simulink model "modello_completo_simulink2020"  (R2020a)
settings: Solver=VariableStepAuto  StartTime=0.0  StopTime=200  RelTol=1e-3
values from neighbouring files (symbols this model uses):
  a = 0.35    [data.m]    (also in geodetic2nedS.m = 6378137)
  a1 = rho * D^4 * alpha1    (= 0.000388302366464)    [data.m]
  a2 = -rho * D^3 * alpha2 * (1 - omega)    (= 0.0037030698432)    [data.m]
  AHRS_bias = [0 0 0]    [data.m]
  AHRS_sample_time = 1/50    (= 0.02)    [data.m]
  AHRS_var = ([1 1 2] * pi/180).^2    [data.m]
  alpha1 = 0.0113    [data.m]
  alpha2 = -0.0091    [data.m]
  c = son2(1)    [Sonar_id.m]    (also in data.m = 0.19)
  current = [seaCurrent; 0; 0; 0]    [data.m]
  D = 0.076    [data.m]
  dead_zone_limit = 31.5    [data.m]
  DVL_sample_t = 1/12    (= 0.0833333333333)    [data.m]
  DVL_var1 = 0.005^2    (= 2.5e-05)    [data.m]
  DVL_var2 = 0.015^2    (= 0.000225)    [data.m]
  DVL_var3 = 0.023^2    (= 0.000529)    [data.m]
  gps_sample_t = 1    [data.m]
  H = eye(3)    [data.m]    (also in navigation_data.m)
  IMU_sample_time = 1/100    (= 0.01)    [data.m]
  initial = []    [data.m]
  INSP = unicode2native(inspectionDirection)    [data.m]
  Ki_bodypos1 = 0    [parametri_PID.m]
  Ki_bodypos2 = 0    [parametri_PID.m]
  Ki_bodypos3 = 0    [parametri_PID.m]
  Ki_bodypos4 = 0    [parametri_PID.m]
  Ki_bodypos5 = 0    [parametri_PID.m]
  Ki_depth1 = 0    [parametri_PID.m]
  Ki_depth2 = 0    [parametri_PID.m]
  Ki_depth3 = 0    [parametri_PID.m]
  Ki_depth4 = 0    [parametri_PID.m]
  Ki_depth5 = 0    [parametri_PID.m]
  Ki_latvel1 = 0    [parametri_PID.m]
  Ki_latvel2 = 0    [parametri_PID.m]
  Ki_latvel3 = 0    [parametri_PID.m]
  Ki_latvel4 = 0    [parametri_PID.m]
  Ki_latvel5 = 0    [parametri_PID.m]
  Ki_P1 = 0    [parametri_PID.m]
  Ki_P2 = 0    [parametri_PID.m]
  Ki_P3 = 0    [parametri_PID.m]
  Ki_P4 = 0    [parametri_PID.m]
  Ki_P5 = 0    [parametri_PID.m]
  Ki_R1 = 0    [parametri_PID.m]
  Ki_R2 = 0    [parametri_PID.m]
  Ki_R3 = 0    [parametri_PID.m]
  Ki_R4 = 0    [parametri_PID.m]
  Ki_R5 = 0    [parametri_PID.m]
  Ki_rel_or1 = 0    [parametri_PID.m]
  Ki_rel_or2 = 0    [parametri_PID.m]
  Ki_rel_or3 = 0    [parametri_PID.m]
  Ki_rel_or4 = 0    [parametri_PID.m]
  Ki_rel_or5 = 0    [parametri_PID.m]
  Ki_reldist1 = 0    [parametri_PID.m]
  Ki_reldist2 = 0    [parametri_PID.m]
  Ki_reldist3 = 0    [parametri_PID.m]
  Ki_reldist4 = 0    [parametri_PID.m]
  Ki_reldist5 = 0    [parametri_PID.m]
  Ki_surge1 = 0    [parametri_PID.m]
  Ki_surge2 = 0    [parametri_PID.m]
  Ki_surge3 = 0    [parametri_PID.m]
  Ki_surge4 = 0    [parametri_PID.m]
  Ki_surge5 = 0    [parametri_PID.m]
  Ki_yaw1 = 0    [parametri_PID.m]
  Ki_yaw2 = 0    [parametri_PID.m]
  Ki_yaw3 = 0    [parametri_PID.m]
  Ki_yaw4 = 0    [parametri_PID.m]
  Ki_yaw5 = 0    [parametri_PID.m]
  Kp_bodypos1 = 0    [parametri_PID.m]
  Kp_bodypos2 = 2    [parametri_PID.m]
  Kp_bodypos3 = 2    [parametri_PID.m]
  Kp_bodypos4 = 2    [parametri_PID.m]
  Kp_bodypos5 = 2    [parametri_PID.m]
  Kp_depth1 = 0    [parametri_PID.m]
  Kp_depth2 = 2    [parametri_PID.m]
  Kp_depth3 = 2    [parametri_PID.m]
  Kp_depth4 = 2    [parametri_PID.m]
  Kp_depth5 = 2    [parametri_PID.m]
  Kp_latvel1 = 0    [parametri_PID.m]
  Kp_latvel2 = 2    [parametri_PID.m]
  Kp_latvel3 = 2    [parametri_PID.m]
  Kp_latvel4 = 2    [parametri_PID.m]
  Kp_latvel5 = 2    [parametri_PID.m]
  Kp_P1 = 0    [parametri_PID.m]
  Kp_P2 = 2    [parametri_PID.m]
  Kp_P3 = 2    [parametri_PID.m]
  Kp_P4 = 2    [parametri_PID.m]
  Kp_P5 = 2    [parametri_PID.m]
  Kp_R1 = 0    [parametri_PID.m]
  Kp_R2 = 2    [parametri_PID.m]
  Kp_R3 = 2    [parametri_PID.m]
  Kp_R4 = 2    [parametri_PID.m]
  Kp_R5 = 2    [parametri_PID.m]
  Kp_rel_or1 = 0    [parametri_PID.m]
  Kp_rel_or2 = 2    [parametri_PID.m]
  Kp_rel_or3 = 2    [parametri_PID.m]
  Kp_rel_or4 = 2    [parametri_PID.m]
  Kp_rel_or5 = 2    [parametri_PID.m]
  Kp_reldist1 = 0    [parametri_PID.m]
  Kp_reldist2 = 2    [parametri_PID.m]
  Kp_reldist3 = 2    [parametri_PID.m]
  Kp_reldist4 = 2    [parametri_PID.m]
  Kp_reldist5 = 2    [parametri_PID.m]
  Kp_surge1 = 0    [parametri_PID.m]
  Kp_surge2 = 2    [parametri_PID.m]
  Kp_surge3 = 2    [parametri_PID.m]
  Kp_surge4 = 2    [parametri_PID.m]
  Kp_surge5 = 2    [parametri_PID.m]
  Kp_yaw1 = 0.6*6    (= 3.6)    [parametri_PID.m]
  Kp_yaw2 = 2    [parametri_PID.m]
  Kp_yaw3 = 2    [parametri_PID.m]
  Kp_yaw4 = 2    [parametri_PID.m]
  Kp_yaw5 = 2    [parametri_PID.m]
  M = M_rb + M_a    [Masse.m]
  M_inv = inv(M)    [Masse.m]
  n_max = 340    [data.m]
  num_cycle = 5    [data.m]    (also in navigation_data.m)
  omega = 0.1    [data.m]
  plot_smpl = 0.1    [data.m]
  ps_sample_t = 0.02    [data.m]
  ps_var = (5000/3)^2    (= 2777777.77778)    [data.m]
  pylonCenter = [ 43.723046 ... (first row only)    [missionB.m]
  ... (+4 more)
undefined symbols (not defined in the file or in its folder): DiscIntNeverNeededParam, s_data
libraries: simulink x3
(part 3 of 5)

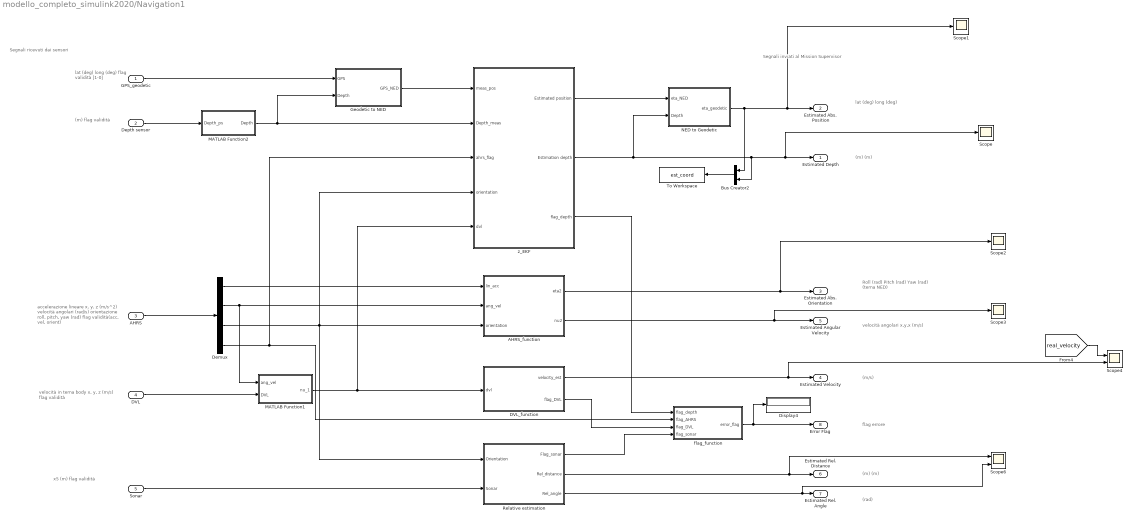
== system modello_completo_simulink2020/Navigation1 ==
  note: (m/s)
  note: (rad)
  note: (m)
      | (m)
  note: (m)
      | flag validità
  note: velocità in terna body x, y, z (m/s)
      | flag validità
  note: Segnali ricevuti dai sensori
  note: flag errore
  note: accelerazione lineare x, y, z (m/s^2)
      | velocità angolari (rad/s)
      | orientazione roll, pitch, yaw (rad)
      | flag validità(acc, vel, orient)
  note: velocità angolari x,y,x (m/s)
  note: lat     (deg)
      |  long  (deg)
  note: (m)
      | (m)
  note: Roll (rad)
      | Pitch (rad)
      | Yaw (rad)
      | (terna NED)
  note: x5
      | (m)
      | flag validità
  note: Segnali inviati al Mission Supervisor
  note: lat     (deg)
      |  long  (deg)
      | flag validità [1-0]
  GPS_geodetic : Inport  PortDimensions=3
  Depth sensor : Inport  Port=2  PortDimensions=2
  AHRS : Inport  Port=3  PortDimensions=12
  DVL : Inport  Port=4  PortDimensions=4
  Sonar : Inport  Port=5
  AHRS_function : MATLAB Function  TreatAsAtomicUnit=on
  Bus Creator2 : BusCreator  Inputs=2
  DVL_function : MATLAB Function  TreatAsAtomicUnit=on
  Demux : Demux  Outputs=[3 3 3 3]
  Display4 : Display
  Geodetic to NED : Subsystem
  MATLAB Function1 : MATLAB Function  TreatAsAtomicUnit=on  SystemSampleTime=DVL_sample_t
  MATLAB Function2 : MATLAB Function  TreatAsAtomicUnit=on
  NED to Geodetic : Subsystem
  Relative estimation : Subsystem
  Scope{,1..3} (4 alike) : Scope
  Scope4 : Scope  NumInputPorts=2
  Scope6 : Scope  NumInputPorts=2
  To Workspace : ToWorkspace  VariableName=est_coord  SampleTime=-1
  flag_function : MATLAB Function  TreatAsAtomicUnit=on  SystemSampleTime=1/200
  z_EKF : Subsystem
  Estimated Depth : Outport
  Estimated Abs. Position : Outport  Port=2
  Estimated Abs. Orientation : Outport  Port=3
  Estimated Velocity : Outport  Port=4
  Estimated Angular Velocity : Outport  Port=5
  Estimated Rel. Distance : Outport  Port=6
  Estimated Rel. Angle : Outport  Port=7
  Error Flag : Outport  Port=8
  wires:
  z_EKF/1(Estimated position) -> NED to Geodetic/1(eta_NED)
  [real_velocity] -> Scope4/1
  Relative estimation/1(Flag_sonar) -> flag_function/4(flag_sonar)
  Bus Creator2/1 -> To Workspace/1
  Demux/4 -> z_EKF/3(ahrs_flag), flag_function/2(flag_AHRS)
  MATLAB Function2/1(Depth) -> Geodetic to NED/2(Depth), z_EKF/2(Depth_meas)
  NED to Geodetic/1(eta_geodetic) -> Bus Creator2/1, Scope1/1, Estimated Abs. Position/1
  z_EKF/3(flag_depth) -> flag_function/1(flag_depth)
  flag_function/1(error_flag) -> Display4/1, Error Flag/1
  AHRS_function/1(eta2) -> Scope2/1, Estimated Abs. Orientation/1
  DVL_function/1(velocity_est) -> Scope4/2, Estimated Velocity/1
  AHRS/1 -> Demux/1
  Sonar/1 -> Relative estimation/2(Sonar)
  Demux/2 -> MATLAB Function1/1(ang_vel), AHRS_function/2(ang_vel)
  Relative estimation/2(Rel_distance) -> Scope6/1, Estimated Rel. Distance/1
  MATLAB Function1/1(nu_1) -> z_EKF/5(dvl), DVL_function/1(dvl)
  Geodetic to NED/1(GPS_NED) -> z_EKF/1(meas_pos)
  z_EKF/2(Estimation depth) -> NED to Geodetic/2(Depth), Bus Creator2/2, Scope/1, Estimated Depth/1
  Relative estimation/3(Rel_angle) -> Scope6/2, Estimated Rel. Angle/1
  GPS_geodetic/1 -> Geodetic to NED/1(GPS)
  DVL_function/2(flag_DVL) -> flag_function/3(flag_DVL)
  Depth sensor/1 -> MATLAB Function2/1(Depth_ps)
  DVL/1 -> MATLAB Function1/2(DVL)
  Demux/3 -> z_EKF/4(orientation), AHRS_function/3(orientation), Relative estimation/1(Orientation)
  AHRS_function/2(nu2) -> Scope3/1, Estimated Angular Velocity/1
  Demux/1 -> AHRS_function/1(lin_acc)

== system modello_completo_simulink2020/Vehicle Model ==
  note: 3x1 (m/s^2),
      | 3x1 (rad/s^2)
  note: 3x1 (m/s),
      | 3x1 (rad/s)
  note: lat (deg)
      | long (deg)
      | prof. (m),
      | roll (rad),
      | pitch (rad),
      | yaw (rad)
  note: 3x1 (m/s),
      | 3x1 (rad/s)
  Desired Thruster Rot. Speed : Inport
  Add : Sum  Inputs=+-
  Constant : Constant  Value=[100; -100; 0; 0; 0; 0; 0]
  Current : Constant  Value=current
  Demux : Demux
  MATLAB Function : MATLAB Function  TreatAsAtomicUnit=on
  Manual (by dashboard sensors) : Subsystem
  Manual Switch : ManualSwitch  CurrentSetting=0
  Manual Switch1 : ManualSwitch
  Model Vehicle : Subsystem
      mask Display: image('$imagefile'); % Use "Edit Image" on toolstrip to change.
  Scope : Scope
  Scope1 : Scope
  Thrusters : Subsystem
      mask Display: image('$imagefile'); % Use "Edit Image" on toolstrip to change.
  Position : Outport
  Velocity_NED : Outport  Port=2
  Acceleration : Outport  Port=3
  Velocity_body : Outport  Port=4
  wires:
  Demux/3 -> Velocity_body/1, Add/2  "ni"
  Model Vehicle/1(Out1) -> Demux/1
  Demux/1 -> Thrusters/2(eta), MATLAB Function/1(eta), Position/1, Scope/1  "eta"
  Desired Thruster Rot. Speed/1 -> Manual Switch/2
  Manual Switch/1 -> Thrusters/1(des rot)
  Current/1 -> MATLAB Function/2(current)
  Demux/2 -> Velocity_NED/1  "eta_dot"
  Demux/4 -> Acceleration/1  "ni_dot"
  MATLAB Function/1(ni_c) -> Model Vehicle/2(ni_current), Add/1
  Add/1 -> Thrusters/3(ni)
  Constant/1 -> Manual Switch/1
  Thrusters/1(tau) -> Manual Switch1/2, Scope1/1
  Manual (by dashboard sensors)/1(y) -> Manual Switch1/1
  Manual Switch1/1 -> Model Vehicle/1(tau)

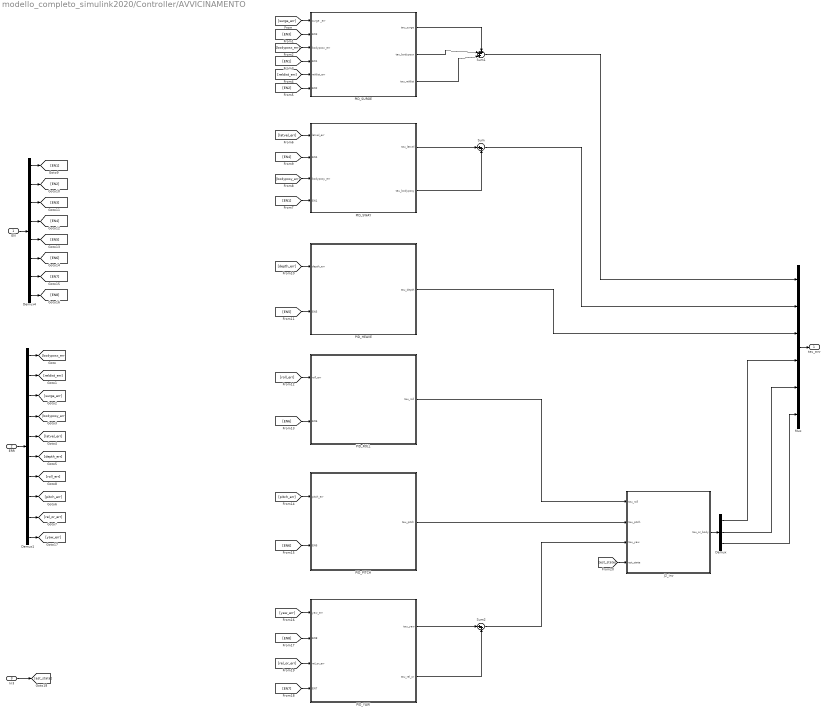
== system modello_completo_simulink2020/Controller/AVVICINAMENTO ==
  EN : Inport
  ERR : Inport  Port=2
  In3 : Inport  Port=3
  Demux : Demux  Outputs=3
  Demux1 : Demux  Outputs=10
  Demux4 : Demux  Outputs=8
  J2_inv : MATLAB Function  TreatAsAtomicUnit=on
  Mux : Mux  Inputs=6
  PID_HEAVE : Subsystem
  PID_PITCH : Subsystem
  "PID_ROLL " : Subsystem
  PID_SURGE : Subsystem
  PID_SWAY : Subsystem
  PID_YAW : Subsystem
  Sum : Sum  Inputs=|++
  Sum1 : Sum  Inputs=+++|
  Sum2 : Sum  Inputs=|++
  tau_avv : Outport
  wires:
  EN/1 -> Demux4/1
  ERR/1 -> Demux1/1
  Demux4/1 -> [EN1]
  Demux4/2 -> [EN2]
  Demux4/3 -> [EN3]
  Demux4/4 -> [EN4]
  Demux4/5 -> [EN5]
  Demux4/6 -> [EN6]
  Demux4/7 -> [EN7]
  Demux4/8 -> [EN8]
  Demux1/1 -> [bodyposx_err]
  Demux1/2 -> [reldist_err]
  Demux1/3 -> [surge_err]
  Demux1/4 -> [bodyposy_err]
  Demux1/5 -> [latvel_err]
  Demux1/6 -> [depth_err]
  Demux1/7 -> [roll_err]
  Demux1/8 -> [pitch_err]
  Demux1/9 -> [rel_or_err]
  Demux1/10 -> [yaw_err]
  [surge_err] -> PID_SURGE/1(surge _err)
  [EN3] -> PID_SURGE/2(EN3)
  [bodyposx_err] -> PID_SURGE/3(bodyposx_err)
  [EN1] -> PID_SURGE/4(EN1)
  [reldist_err] -> PID_SURGE/5(reldist_err)
  [EN2] -> PID_SURGE/6(EN2)
  [latvel_err] -> PID_SWAY/1(latvel_err)
  [bodyposy_err] -> PID_SWAY/3(bodyposy_err)
  [depth_err] -> PID_HEAVE/1(depth_err)
  [roll_err] -> "PID_ROLL "/1(roll_err)
  [pitch_err] -> PID_PITCH/1(pitch_err)
  [EN6] -> PID_PITCH/2(EN6)
  [yaw_err] -> PID_YAW/1(yaw_err)
  [EN4] -> PID_SWAY/2(EN4)
  [EN1] -> PID_SWAY/4(EN1)
  [EN5] -> PID_HEAVE/2(EN5)
  [EN6] -> "PID_ROLL "/2(EN6)
  [EN8] -> PID_YAW/2("EN8 ")
  [EN7] -> PID_YAW/4(EN7)
  [rel_or_err] -> PID_YAW/3(rel_or_err)
  PID_HEAVE/1(tau_depth) -> Mux/3
  PID_SURGE/1(tau_surge) -> Sum1/1
  Mux/1 -> tau_avv/1
  Sum1/1 -> Mux/1
  Sum/1 -> Mux/2
  PID_YAW/1(tau_yaw) -> Sum2/1
  PID_SWAY/2(tau_bodyposy) -> Sum/2
  PID_SURGE/3(tau_reldist) -> Sum1/3
  PID_SURGE/2(tau_bodyposx) -> Sum1/2
  PID_YAW/2(tau_rel_or) -> Sum2/2
  PID_SWAY/1(tau_latvel) -> Sum/1
  Demux/2 -> Mux/5
  PID_PITCH/1(tau_pitch) -> J2_inv/2(tau_pitch)
  J2_inv/1(tau_or_body) -> Demux/1
  Demux/3 -> Mux/6
  "PID_ROLL "/1(tau_roll) -> J2_inv/1(tau_roll)
  Demux/1 -> Mux/4
  [est_state] -> J2_inv/4(est_state)
  Sum2/1 -> J2_inv/3(tau_yaw)
  In3/1 -> [est_state]

== system modello_completo_simulink2020/Controller/GEODETIC2NED2 ==
  Estimated Abs. Postion : Inport  Unit=deg  PortDimensions=2
  GEODETIC2NED1 : Subsystem
  Out1 : Outport
  wires:
  GEODETIC2NED1/1(Out1) -> Out1/1
  Estimated Abs. Postion/1 -> GEODETIC2NED1/1(In1)

== system modello_completo_simulink2020/Controller/GEODETIC2NED3 ==
  In1 : Inport
  Demux2 : Demux  Outputs=2
  GEODETIC2NED : Subsystem
  Out1 : Outport
  wires:
  Demux2/2 -> GEODETIC2NED/2(lon)
  GEODETIC2NED/1(Out1) -> Out1/1
  Demux2/1 -> GEODETIC2NED/1(lat)
  In1/1 -> Demux2/1

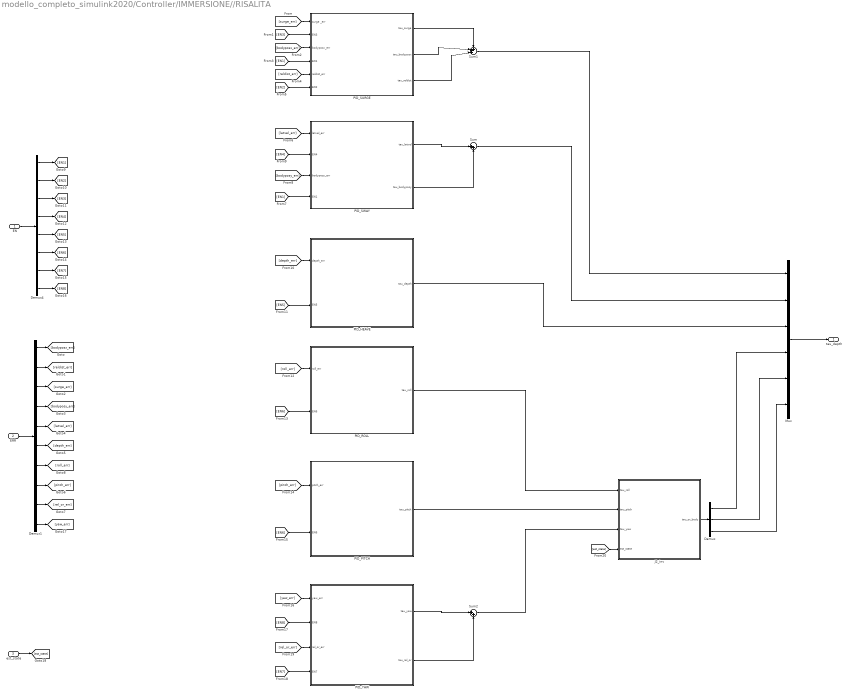
== system modello_completo_simulink2020/Controller/IMMERSIONE//RISALITA ==
  EN : Inport
  ERR : Inport  Port=2
  est_state : Inport  Port=3
  Demux : Demux  Outputs=3
  Demux1 : Demux  Outputs=10
  Demux4 : Demux  Outputs=8
  J2_inv : MATLAB Function  TreatAsAtomicUnit=on
  Mux : Mux  Inputs=6
  PID_HEAVE : Subsystem
  PID_PITCH : Subsystem
  "PID_ROLL " : Subsystem
  PID_SURGE : Subsystem
  PID_SWAY : Subsystem
  PID_YAW : Subsystem
  Sum : Sum  Inputs=|++
  Sum1 : Sum  Inputs=+++|
  Sum2 : Sum  Inputs=|++
  tau_depth : Outport
  wires:
  EN/1 -> Demux4/1
  ERR/1 -> Demux1/1
  Demux4/1 -> [EN1]
  Demux4/2 -> [EN2]
  Demux4/3 -> [EN3]
  Demux4/4 -> [EN4]
  Demux4/5 -> [EN5]
  Demux4/6 -> [EN6]
  Demux4/7 -> [EN7]
  Demux4/8 -> [EN8]
  Demux1/1 -> [bodyposx_err]
  Demux1/2 -> [reldist_err]
  Demux1/3 -> [surge_err]
  Demux1/4 -> [bodyposy_err]
  Demux1/5 -> [latvel_err]
  Demux1/6 -> [depth_err]
  Demux1/7 -> [roll_err]
  Demux1/8 -> [pitch_err]
  Demux1/9 -> [rel_or_err]
  Demux1/10 -> [yaw_err]
  [surge_err] -> PID_SURGE/1(surge _err)
  [EN3] -> PID_SURGE/2(EN3)
  [bodyposx_err] -> PID_SURGE/3(bodyposx_err)
  [EN1] -> PID_SURGE/4(EN1)
  [reldist_err] -> PID_SURGE/5(reldist_err)
  [EN2] -> PID_SURGE/6(EN2)
  [latvel_err] -> PID_SWAY/1(latvel_err)
  [bodyposy_err] -> PID_SWAY/3(bodyposy_err)
  [depth_err] -> PID_HEAVE/1(depth_err)
  [roll_err] -> "PID_ROLL "/1(roll_err)
  [pitch_err] -> PID_PITCH/1(pitch_err)
  [EN6] -> PID_PITCH/2(EN6)
  [yaw_err] -> PID_YAW/1(yaw_err)
  [EN4] -> PID_SWAY/2(EN4)
  [EN1] -> PID_SWAY/4(EN1)
  [EN5] -> PID_HEAVE/2(EN5)
  [EN6] -> "PID_ROLL "/2(EN6)
  [EN8] -> PID_YAW/2("EN8 ")
  [EN7] -> PID_YAW/4(EN7)
  [rel_or_err] -> PID_YAW/3(rel_or_err)
  PID_HEAVE/1(tau_depth) -> Mux/3
  PID_SURGE/1(tau_surge) -> Sum1/1
  Mux/1 -> tau_depth/1
  Sum1/1 -> Mux/1
  Sum/1 -> Mux/2
  PID_YAW/1(tau_yaw) -> Sum2/1
  PID_SWAY/2(tau_bodyposy) -> Sum/2
  PID_SURGE/3(tau_reldist) -> Sum1/3
  PID_SURGE/2(tau_bodyposx) -> Sum1/2
  PID_YAW/2(tau_rel_or) -> Sum2/2
  PID_SWAY/1(tau_latvel) -> Sum/1
  Demux/2 -> Mux/5
  [est_state] -> J2_inv/4(est_state)
  "PID_ROLL "/1(tau_roll) -> J2_inv/1(tau_roll)
  Demux/3 -> Mux/6
  Demux/1 -> Mux/4
  PID_PITCH/1(tau_pitch) -> J2_inv/2(tau_pitch)
  Sum2/1 -> J2_inv/3(tau_yaw)
  J2_inv/1(tau_or_body) -> Demux/1
  est_state/1 -> [est_state]

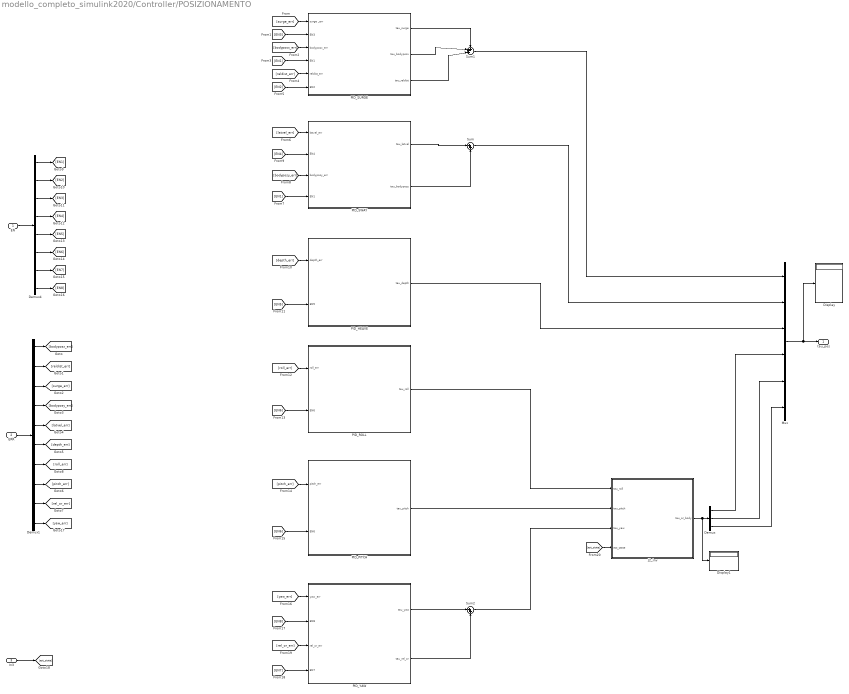
== system modello_completo_simulink2020/Controller/POSIZIONAMENTO ==
  EN : Inport
  ERR : Inport  Port=2
  In3 : Inport  Port=3
  Demux : Demux  Outputs=3
  Demux1 : Demux  Outputs=10
  Demux4 : Demux  Outputs=8
  Display : Display
  Display1 : Display
  J2_inv : MATLAB Function  TreatAsAtomicUnit=on
  Mux : Mux  Inputs=6
  PID_HEAVE : Subsystem
  PID_PITCH : Subsystem
  "PID_ROLL " : Subsystem
  PID_SURGE : Subsystem
  PID_SWAY : Subsystem
  PID_YAW : Subsystem
  Sum : Sum  Inputs=|++
  Sum1 : Sum  Inputs=+++|
  Sum2 : Sum  Inputs=|++
  tau_pos : Outport
  wires:
  PID_SWAY/1(tau_latvel) -> Sum/1
  PID_YAW/2(tau_rel_or) -> Sum2/2
  PID_SURGE/2(tau_bodyposx) -> Sum1/2
  PID_SURGE/3(tau_reldist) -> Sum1/3
  PID_SWAY/2(tau_bodyposy) -> Sum/2
  PID_YAW/1(tau_yaw) -> Sum2/1
  Sum/1 -> Mux/2
  Sum1/1 -> Mux/1
  Mux/1 -> Display/1, tau_pos/1
  PID_SURGE/1(tau_surge) -> Sum1/1
  PID_HEAVE/1(tau_depth) -> Mux/3
  [rel_or_err] -> PID_YAW/3(rel_or_err)
  [EN7] -> PID_YAW/4(EN7)
  [EN8] -> PID_YAW/2("EN8 ")
  [EN6] -> "PID_ROLL "/2(EN6)
  [EN5] -> PID_HEAVE/2(EN5)
  [EN1] -> PID_SWAY/4(EN1)
  [EN4] -> PID_SWAY/2(EN4)
  [yaw_err] -> PID_YAW/1(yaw_err)
  [EN6] -> PID_PITCH/2(EN6)
  [pitch_err] -> PID_PITCH/1(pitch_err)
  [roll_err] -> "PID_ROLL "/1(roll_err)
  [depth_err] -> PID_HEAVE/1(depth_err)
  [bodyposy_err] -> PID_SWAY/3(bodyposy_err)
  [latvel_err] -> PID_SWAY/1(latvel_err)
  [EN2] -> PID_SURGE/6(EN2)
  [reldist_err] -> PID_SURGE/5(reldist_err)
  [EN1] -> PID_SURGE/4(EN1)
  [bodyposx_err] -> PID_SURGE/3(bodyposx_err)
  [EN3] -> PID_SURGE/2(EN3)
  [surge_err] -> PID_SURGE/1(surge _err)
  Demux1/10 -> [yaw_err]
  Demux1/9 -> [rel_or_err]
  Demux1/8 -> [pitch_err]
  Demux1/7 -> [roll_err]
  Demux1/6 -> [depth_err]
  Demux1/5 -> [latvel_err]
  Demux1/4 -> [bodyposy_err]
  Demux1/3 -> [surge_err]
  Demux1/2 -> [reldist_err]
  Demux1/1 -> [bodyposx_err]
  Demux4/8 -> [EN8]
  Demux4/7 -> [EN7]
  Demux4/6 -> [EN6]
  Demux4/5 -> [EN5]
  Demux4/4 -> [EN4]
  Demux4/3 -> [EN3]
  Demux4/2 -> [EN2]
  Demux4/1 -> [EN1]
  ERR/1 -> Demux1/1
  EN/1 -> Demux4/1
  In3/1 -> [est_state]
  [est_state] -> J2_inv/4(est_state)
  "PID_ROLL "/1(tau_roll) -> J2_inv/1(tau_roll)
  PID_PITCH/1(tau_pitch) -> J2_inv/2(tau_pitch)
  Sum2/1 -> J2_inv/3(tau_yaw)
  J2_inv/1(tau_or_body) -> Display1/1, Demux/1
  Demux/1 -> Mux/4
  Demux/2 -> Mux/5
  Demux/3 -> Mux/6

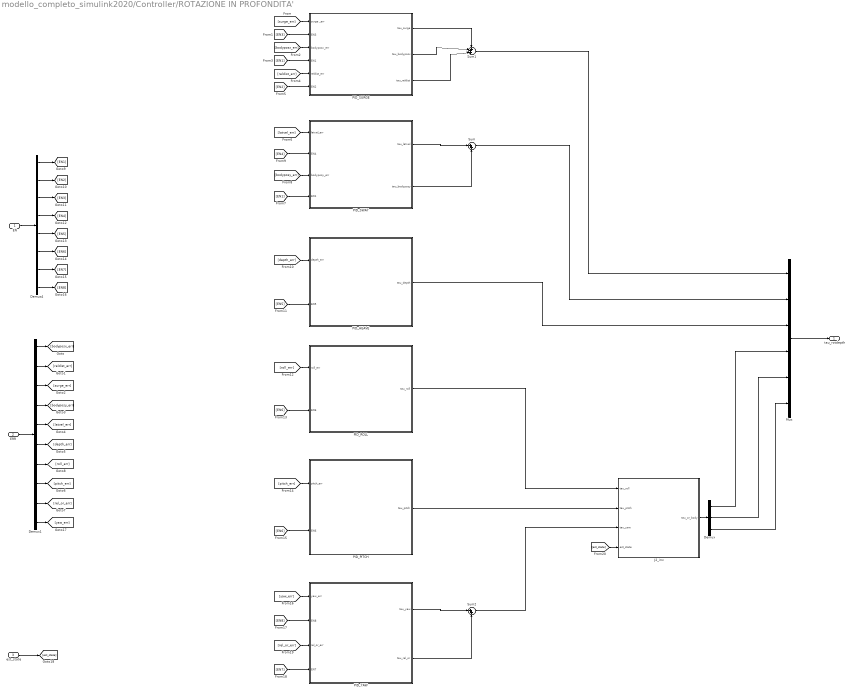
== system modello_completo_simulink2020/Controller/ROTAZIONE IN PROFONDITA' ==
  EN : Inport
  ERR : Inport  Port=2
  est_state : Inport  Port=3
  Demux : Demux  Outputs=3
  Demux1 : Demux  Outputs=10
  Demux4 : Demux  Outputs=8
  J2_inv : MATLAB Function  TreatAsAtomicUnit=on
  Mux : Mux  Inputs=6
  PID_HEAVE : Subsystem
  PID_PITCH : Subsystem
  "PID_ROLL " : Subsystem
  PID_SURGE : Subsystem
  PID_SWAY : Subsystem
  PID_YAW : Subsystem
  Sum : Sum  Inputs=|++
  Sum1 : Sum  Inputs=+++|
  Sum2 : Sum  Inputs=|++
  tau_rotdepth : Outport
  wires:
  EN/1 -> Demux4/1
  ERR/1 -> Demux1/1
  Demux4/1 -> [EN1]
  Demux4/2 -> [EN2]
  Demux4/3 -> [EN3]
  Demux4/4 -> [EN4]
  Demux4/5 -> [EN5]
  Demux4/6 -> [EN6]
  Demux4/7 -> [EN7]
  Demux4/8 -> [EN8]
  Demux1/1 -> [bodyposx_err]
  Demux1/2 -> [reldist_err]
  Demux1/3 -> [surge_err]
  Demux1/4 -> [bodyposy_err]
  Demux1/5 -> [latvel_err]
  Demux1/6 -> [depth_err]
  Demux1/7 -> [roll_err]
  Demux1/8 -> [pitch_err]
  Demux1/9 -> [rel_or_err]
  Demux1/10 -> [yaw_err]
  [surge_err] -> PID_SURGE/1(surge _err)
  [EN3] -> PID_SURGE/2(EN3)
  [bodyposx_err] -> PID_SURGE/3(bodyposx_err)
  [EN1] -> PID_SURGE/4(EN1)
  [reldist_err] -> PID_SURGE/5(reldist_err)
  [EN2] -> PID_SURGE/6(EN2)
  [latvel_err] -> PID_SWAY/1(latvel_err)
  [bodyposy_err] -> PID_SWAY/3(bodyposy_err)
  [depth_err] -> PID_HEAVE/1(depth_err)
  [roll_err] -> "PID_ROLL "/1(roll_err)
  [pitch_err] -> PID_PITCH/1(pitch_err)
  [EN6] -> PID_PITCH/2(EN6)
  [yaw_err] -> PID_YAW/1(yaw_err)
  [EN4] -> PID_SWAY/2(EN4)
  [EN1] -> PID_SWAY/4(EN1)
  [EN5] -> PID_HEAVE/2(EN5)
  [EN6] -> "PID_ROLL "/2(EN6)
  [EN8] -> PID_YAW/2("EN8 ")
  [EN7] -> PID_YAW/4(EN7)
  [rel_or_err] -> PID_YAW/3(rel_or_err)
  PID_HEAVE/1(tau_depth) -> Mux/3
  PID_SURGE/1(tau_surge) -> Sum1/1
  Mux/1 -> tau_rotdepth/1
  Sum1/1 -> Mux/1
  Sum/1 -> Mux/2
  PID_YAW/1(tau_yaw) -> Sum2/1
  PID_SWAY/2(tau_bodyposy) -> Sum/2
  PID_SURGE/3(tau_reldist) -> Sum1/3
  PID_SURGE/2(tau_bodyposx) -> Sum1/2
  PID_YAW/2(tau_rel_or) -> Sum2/2
  PID_SWAY/1(tau_latvel) -> Sum/1
  Demux/1 -> Mux/4
  Sum2/1 -> J2_inv/3(tau_yaw)
  Demux/3 -> Mux/6
  "PID_ROLL "/1(tau_roll) -> J2_inv/1(tau_roll)
  Demux/2 -> Mux/5
  [est_state] -> J2_inv/4(est_state)
  PID_PITCH/1(tau_pitch) -> J2_inv/2(tau_pitch)
  J2_inv/1(tau_or_body) -> Demux/1
  est_state/1 -> [est_state]

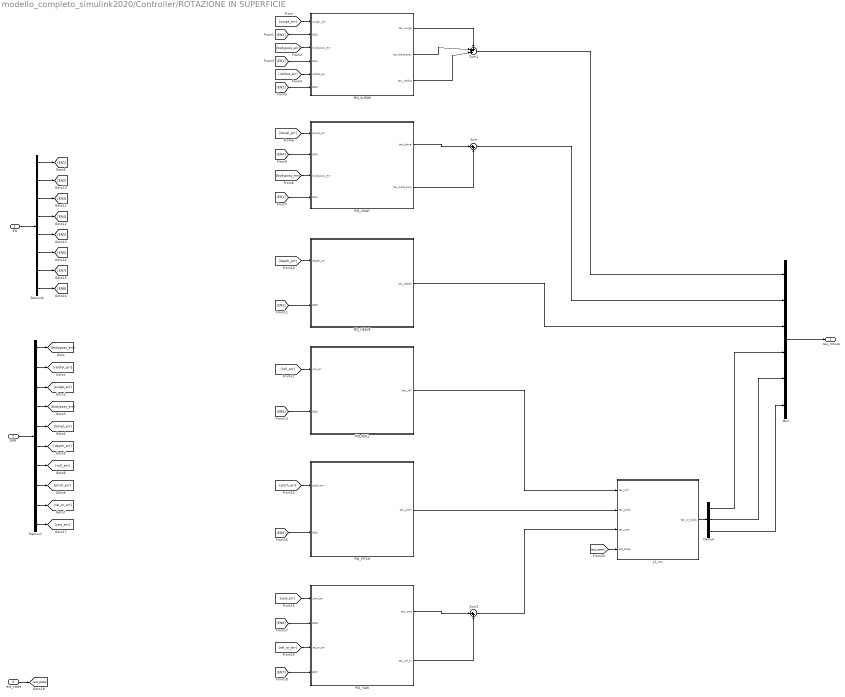
== system modello_completo_simulink2020/Controller/ROTAZIONE IN SUPERFICIE ==
  EN : Inport
  ERR : Inport  Port=2
  est_state : Inport  Port=3
  Demux : Demux  Outputs=3
  Demux1 : Demux  Outputs=10
  Demux4 : Demux  Outputs=8
  J2_inv : MATLAB Function  TreatAsAtomicUnit=on
  Mux : Mux  Inputs=6
  PID_HEAVE : Subsystem
  PID_PITCH : Subsystem
  "PID_ROLL " : Subsystem
  PID_SURGE : Subsystem
  PID_SWAY : Subsystem
  PID_YAW : Subsystem
  Sum : Sum  Inputs=|++
  Sum1 : Sum  Inputs=+++|
  Sum2 : Sum  Inputs=|++
  tau_rotsup : Outport
  wires:
  EN/1 -> Demux4/1
  ERR/1 -> Demux1/1
  Demux4/1 -> [EN1]
  Demux4/2 -> [EN2]
  Demux4/3 -> [EN3]
  Demux4/4 -> [EN4]
  Demux4/5 -> [EN5]
  Demux4/6 -> [EN6]
  Demux4/7 -> [EN7]
  Demux4/8 -> [EN8]
  Demux1/1 -> [bodyposx_err]
  Demux1/2 -> [reldist_err]
  Demux1/3 -> [surge_err]
  Demux1/4 -> [bodyposy_err]
  Demux1/5 -> [latvel_err]
  Demux1/6 -> [depth_err]
  Demux1/7 -> [roll_err]
  Demux1/8 -> [pitch_err]
  Demux1/9 -> [rel_or_err]
  Demux1/10 -> [yaw_err]
  [surge_err] -> PID_SURGE/1(surge _err)
  [EN3] -> PID_SURGE/2(EN3)
  [bodyposx_err] -> PID_SURGE/3(bodyposx_err)
  [EN1] -> PID_SURGE/4(EN1)
  [reldist_err] -> PID_SURGE/5(reldist_err)
  [EN2] -> PID_SURGE/6(EN2)
  [latvel_err] -> PID_SWAY/1(latvel_err)
  [bodyposy_err] -> PID_SWAY/3(bodyposy_err)
  [depth_err] -> PID_HEAVE/1(depth_err)
  [roll_err] -> "PID_ROLL "/1(roll_err)
  [pitch_err] -> PID_PITCH/1(pitch_err)
  [EN6] -> PID_PITCH/2(EN6)
  [yaw_err] -> PID_YAW/1(yaw_err)
  [EN4] -> PID_SWAY/2(EN4)
  [EN1] -> PID_SWAY/4(EN1)
  [EN5] -> PID_HEAVE/2(EN5)
  [EN6] -> "PID_ROLL "/2(EN6)
  [EN8] -> PID_YAW/2("EN8 ")
  [EN7] -> PID_YAW/4(EN7)
  [rel_or_err] -> PID_YAW/3(rel_or_err)
  PID_HEAVE/1(tau_depth) -> Mux/3
  PID_SURGE/1(tau_surge) -> Sum1/1
  Mux/1 -> tau_rotsup/1
  Sum1/1 -> Mux/1
  Sum/1 -> Mux/2
  PID_YAW/1(tau_yaw) -> Sum2/1
  PID_SWAY/2(tau_bodyposy) -> Sum/2
  PID_SURGE/3(tau_reldist) -> Sum1/3
  PID_SURGE/2(tau_bodyposx) -> Sum1/2
  PID_YAW/2(tau_rel_or) -> Sum2/2
  PID_SWAY/1(tau_latvel) -> Sum/1
  J2_inv/1(tau_or_body) -> Demux/1
  "PID_ROLL "/1(tau_roll) -> J2_inv/1(tau_roll)
  Demux/3 -> Mux/6
  Demux/1 -> Mux/4
  PID_PITCH/1(tau_pitch) -> J2_inv/2(tau_pitch)
  [est_state] -> J2_inv/4(est_state)
  Demux/2 -> Mux/5
  Sum2/1 -> J2_inv/3(tau_yaw)
  est_state/1 -> [est_state]

== system modello_completo_simulink2020/Controller/SATURATION ==
  In2 : Inport
  Saturation3 : Saturate  UpperLimit=45  LowerLimit=-45
  Out2 : Outport
  wires:
  In2/1 -> Saturation3/1
  Saturation3/1 -> Out2/1

== system modello_completo_simulink2020/Controller/T2n ==
  Tdes : Inport
  MATLAB Function : MATLAB Function  TreatAsAtomicUnit=on
  n : Outport  Unit=rad/s  PortDimensions=7
  wires:
  Tdes/1 -> MATLAB Function/1(Tdes)
  MATLAB Function/1(n) -> n/1

== system modello_completo_simulink2020/Controller/Tau2T ==
  tau_pos : Inport
  tau_avv : Inport  Port=2
  tau_rotsup : Inport  Port=3
  tau_depth : Inport  Port=4
  tau_rotdepth : Inport  Port=5
  In6 : Inport  Port=6
  Constant : Constant  Value=101
  Data Store Read : DataStoreRead  DataStoreName=current_state  SampleTime=0.1
  Display : Display
  Display1 : Display
  Manual Switch : ManualSwitch  CurrentSetting=0
  Tau2T : MATLAB Function  TreatAsAtomicUnit=on
  Tau_des ENABLE : MATLAB Function  TreatAsAtomicUnit=on
  Tdes : Outport
  wires:
  Tau2T/1(T) -> Display1/1, Tdes/1
  tau_pos/1 -> Tau_des ENABLE/2(tau1)
  tau_avv/1 -> Tau_des ENABLE/3(tau2)
  tau_rotsup/1 -> Tau_des ENABLE/4(tau3)
  tau_depth/1 -> Tau_des ENABLE/5(tau4)
  tau_rotdepth/1 -> Tau_des ENABLE/6(tau5)
  Tau_des ENABLE/1(tau_des) -> Display/1, Tau2T/1(tau_des)
  Constant/1 -> Manual Switch/1
  Manual Switch/1 -> Tau_des ENABLE/1(STATE)
  In6/1 -> Manual Switch/2

== system modello_completo_simulink2020/Env. & Sensor Model1/AHRS SENSOR ==
  note: AHRS
      |
      | Dynamic Accuracy (Heading):   2.0° RMS
      | Dynamic Accuracy (Pitch/Roll): 1.0° RMS
  note: Output Rate (IMU Data): 800 Hz
  note: Resolution:
  note: 0.02		      	 °
      | 0.3491 * 10-3 rad
  note: 0.05				°
      | 0,8727 * 10^-3	rad
  note: 0,0015 Gauss
  note: Vectornav VN-100 IMU/AHRS
  note: IMU
  note: 0.05			    mg
      | 0.4905 * 10^-3  m/s^2
  note: Output Rate (Attitude Data): 400 Hz
  ni_1 : Inport  SampleTime=IMU_sample_time
  ni_1_dot : Inport  Port=2  SampleTime=IMU_sample_time
  ni_2 : Inport  Port=3  SampleTime=IMU_sample_time
  eta_2 : Inport  Port=4  SampleTime=AHRS_sample_time
  eta_2_dot : Inport  Port=5  SampleTime=IMU_sample_time
  "   " : MATLAB Function  TreatAsAtomicUnit=on
  ACC : Constant
  AHRS2 : Constant
  Accelerometer : Subsystem
  Bus Creator : BusCreator  Inputs=3
  GYRO : Constant
  Gyroscope : Subsystem
  Magnetometer : Subsystem
  Noise : Gain
  Quantizer : Quantizer  QuantizationInterval=Resolution_acc
  Quantizer1 : Quantizer  QuantizationInterval=Resolution_gyro
  Quantizer2 : Quantizer  QuantizationInterval=Resolution_magn
  Quantizer3 : Quantizer  QuantizationInterval=Resolution_AHRS
  Random Number : RandomNumber  Mean=AHRS_bias  Variance=AHRS_var  Seed=[232 342 202]  SampleTime=AHRS_sample_time
  Scope : Scope
  Sum : Sum  Inputs=|++
  Output8 : Outport  SampleTime=IMU_sample_time
  Output9 : Outport  Port=2  SampleTime=IMU_sample_time
  Output10 : Outport  Port=3  SampleTime=AHRS_sample_time
  Output : Outport  Port=4  SampleTime=AHRS_sample_time
  wires:
  "   "/2(ang_vel) -> Gyroscope/1(In1)
  Gyroscope/1(ang_vel) -> Quantizer1/1
  ni_1/1 -> "   "/1(ni_1)
  eta_2/1 -> Sum/2, "   "/4(eta_2)
  ni_2/1 -> "   "/3(ni_2)
  Quantizer2/1 -> Scope/1  "AHRS"
  Quantizer1/1 -> Output9/1  "Gyro"
  Accelerometer/1(lin_acc) -> Quantizer/1
  ni_1_dot/1 -> "   "/2(ni_1_dot)
  Sum/1 -> Quantizer3/1
  "   "/1(lin_acc) -> Accelerometer/1(In1)
  Quantizer/1 -> Output8/1  "Acc"
  eta_2_dot/1 -> "   "/5(eta_2_dot)
  Random Number/1 -> Noise/1
  "   "/3(m) -> Magnetometer/1(In1)
  Magnetometer/1(m) -> Quantizer2/1
  Quantizer3/1 -> Output10/1  "AHRS"
  ACC/1 -> Bus Creator/1
  GYRO/1 -> Bus Creator/2
  AHRS2/1 -> Bus Creator/3
  Bus Creator/1 -> Output/1
  Noise/1 -> Sum/1

== system modello_completo_simulink2020/Env. & Sensor Model1/DVL SENSOR ==
  By model2 : Inport  SampleTime=DVL_sample_t
  AND1 : Logic  IconShape=distinctive  AllPortsSameDT=off  OutDataTypeStr=boolean
  DVL : Constant
  Data Type Conversion : DataTypeConversion  OutDataTypeStr=double
  Demux : Demux  Outputs=3
  MATLAB Function : MATLAB Function  TreatAsAtomicUnit=on
  MATLAB Function2 : MATLAB Function  TreatAsAtomicUnit=on
  Quantizer : Quantizer  QuantizationInterval=DVL_resol
  Selector9 : Selector  InputPortWidth=6  IndexOptions=Index vector (dialog)  Indices=[1 2 3]  OutputSizes=1
  Subsystem : Subsystem
  Subsystem1 : Subsystem
  Subsystem2 : Subsystem
  Sum1 : Sum  Inputs=|++
  Sum2 : Sum  Inputs=|++
  Sum3 : Sum  Inputs=|++
  Vector Concatenate : Concatenate  NumInputs=3
  v_sens1 : Outport  SampleTime=DVL_sample_t
  flag_DVL : Outport  Port=2  SampleTime=DVL_sample_t
  wires:
  MATLAB Function2/1(flag) -> AND1/1
  DVL/1 -> AND1/2
  AND1/1 -> Data Type Conversion/1
  Demux/1 -> Sum1/1, Subsystem/1(In1)  "Vx"
  Subsystem/1(Out1) -> Sum1/2
  Demux/2 -> Sum2/1, Subsystem1/1(In1)  "Vy"
  Subsystem1/1(Out1) -> Sum2/2
  Demux/3 -> Sum3/1, Subsystem2/1(In1)  "Vz"
  Subsystem2/1(Out1) -> Sum3/2
  Sum2/1 -> Vector Concatenate/2  "Vy"
  Sum1/1 -> Vector Concatenate/1  "Vx"
  Sum3/1 -> Vector Concatenate/3  "Vz"
  Vector Concatenate/1 -> Quantizer/1
  By model2/1 -> MATLAB Function/1(ni), Selector9/1
  Quantizer/1 -> v_sens1/1
  Data Type Conversion/1 -> flag_DVL/1
  Selector9/1 -> MATLAB Function2/1(v)
  MATLAB Function/1(niDVL) -> Demux/1

== system modello_completo_simulink2020/Env. & Sensor Model1/GPS SENSOR ==
  note: Copernicus II DIP
  note: Control state sensors. 1:enabled, 0:disabled
  "[x, y, z] [m]" : Inport  SampleTime=gps_sample_t
  eta : Inport  Port=2
  Add noiose : Subsystem
  Control state : Subsystem
  Demux : Demux  Outputs=3
  For dashboard : Subsystem
  MATLAB Function : MATLAB Function  TreatAsAtomicUnit=on
  NED2Geodetic : MATLAB Function  TreatAsAtomicUnit=on
  Threshold : MATLAB Function  TreatAsAtomicUnit=on
  Zero-Order Hold : ZeroOrderHold  SampleTime=gps_sample_t
  Lat e Lon Measure [deg] : Outport
  Flag enable gps : Outport  Port=2
  wires:
  Threshold/2(x_out) -> MATLAB Function/1(x)  "x real"
  Threshold/3(y_out) -> MATLAB Function/2(y)  "y real"
  Threshold/1(depth) -> NED2Geodetic/1(depth)  "Depth"
  Add noiose/1(Out1) -> NED2Geodetic/2(u)  "x and y plus noise"
  Threshold/4(flag_enable_gps) -> Control state/1(In1)  "flag enable gps"
  Control state/1(Flag enable gps) -> NED2Geodetic/3(enableGps), Flag enable gps/1
  NED2Geodetic/1(data_GDT) -> Zero-Order Hold/1
  "[x, y, z] [m]"/1 -> Demux/1
  Demux/1 -> Threshold/1(x_in)
  Demux/2 -> Threshold/2(y_in)
  Demux/3 -> Threshold/3(h_in)
  Zero-Order Hold/1 -> For dashboard/1((deg/deg)), Lat e Lon Measure [deg]/1  "(deg/deg)"
  eta/1 -> MATLAB Function/3(eta)
  MATLAB Function/2(yS) -> Add noiose/2(In2)
  MATLAB Function/1(xS) -> Add noiose/1(In1)

== system modello_completo_simulink2020/Env. & Sensor Model1/Pressure sensor ==
  h : Inport  SampleTime=ps_sample_t
  orient : Inport  Port=2
  DEPTH MEASUREMENT : Constant
  MATLAB Function2 : MATLAB Function  TreatAsAtomicUnit=on
  MATLAB Function3 : MATLAB Function  TreatAsAtomicUnit=on
  Noise : Gain
  Quantizer1 : Quantizer  QuantizationInterval=ps_resol  LinearizeAsGain=off
  Random Number1 : RandomNumber  Variance=ps_var  SampleTime=ps_sample_t
  Sum1 : Sum  Inputs=|++
  Zero-Order Hold : ZeroOrderHold  SampleTime=ps_sample_t
  Output1 : Outport  SampleTime=ps_sample_t
  Output7 : Outport  Port=2
  wires:
  DEPTH MEASUREMENT/1 -> Output7/1
  Random Number1/1 -> Noise/1
  MATLAB Function2/1(p) -> Sum1/1
  MATLAB Function3/1(h) -> Zero-Order Hold/1
  Sum1/1 -> Quantizer1/1
  Quantizer1/1 -> MATLAB Function3/2(p)
  h/1 -> MATLAB Function2/1(h)
  Zero-Order Hold/1 -> Output1/1  "Depth"
  orient/1 -> MATLAB Function3/1(orient)
  Noise/1 -> Sum1/2

== system modello_completo_simulink2020/Env. & Sensor Model1/Sonar sensor ==
  Position (m) (NED) : Inport  SampleTime=s_data.smpl
  Orientation (rad) : Inport  Port=2  SampleTime=s_data.smpl
  Demux : Demux  Outputs=3
  Demux1 : Demux  Outputs=3
  For dashboard : Subsystem
  Gain : Gain  Gain=8*ones(5,1)  Multiplication=Matrix(K*u)
  MATLAB Function : MATLAB Function  TreatAsAtomicUnit=on
  MATLAB Function1 : MATLAB Function  TreatAsAtomicUnit=on
  Noises : Subsystem
  Quantizer : Quantizer  QuantizationInterval=s_data.res
  SONAR : Constant  Value=0
  Sum : Sum  Inputs=++|
  Sonar : Outport
  Flag : Outport  Port=2
  Son : Outport  Port=3
  wires:
  MATLAB Function/1(s) -> MATLAB Function1/1(s_in)
  MATLAB Function1/1(s_out) -> Sum/2
  Noises/1(Noises) -> Sum/1
  Position (m) (NED)/1 -> Demux/1
  Demux/1 -> MATLAB Function/1(xNorth)
  Demux/2 -> MATLAB Function/2(yEast)
  Demux/3 -> MATLAB Function/3(zDown), MATLAB Function1/2(depth)
  Demux1/3 -> MATLAB Function/6(yaw)
  Demux1/2 -> MATLAB Function/5(pitch)
  Demux1/1 -> MATLAB Function/4(roll)
  Orientation (rad)/1 -> Demux1/1
  SONAR/1 -> Gain/1
  Gain/1 -> MATLAB Function1/3(error)
  Quantizer/1 -> For dashboard/1(In1), Sonar/1
  MATLAB Function1/2(flag) -> Flag/1
  Sum/1 -> Quantizer/1
  MATLAB Function/2(son) -> Son/1

== system modello_completo_simulink2020/Navigation1/Geodetic to NED ==
  GPS : Inport
  Depth : Inport  Port=2
  Demux : Demux  Outputs=2
  Demux1 : Demux  Outputs=[2 1]
  Gain1 : Gain  Gain=pi/180
  MATLAB Function2 : MATLAB Function  TreatAsAtomicUnit=on
  Terminator : Terminator
  GPS_NED : Outport
  wires:
  Demux1/2 -> MATLAB Function2/2(GPS_flag)
  MATLAB Function2/1(GPS_NED) -> GPS_NED/1
  GPS/1 -> Demux1/1
  Demux1/1 -> Gain1/1
  Gain1/1 -> MATLAB Function2/1(GPS_geodetic)
  Depth/1 -> Demux/1
  Demux/1 -> MATLAB Function2/3(depth)
  Demux/2 -> Terminator/1

== system modello_completo_simulink2020/Navigation1/NED to Geodetic ==
  eta_NED : Inport
  Depth : Inport  Port=2
  Gain : Gain  Gain=180/pi
  MATLAB Function1 : MATLAB Function  TreatAsAtomicUnit=on
  eta_geodetic : Outport  PortDimensions=2
  wires:
  Gain/1 -> eta_geodetic/1
  eta_NED/1 -> MATLAB Function1/1(eta_NED)
  MATLAB Function1/1(eta_geodetic) -> Gain/1
  Depth/1 -> MATLAB Function1/2(depth)

== system modello_completo_simulink2020/Navigation1/Relative estimation ==
  Orientation : Inport
  Sonar : Inport  Port=2
  Demux : Demux  Outputs=[5 5]
  Demux1 : Demux  Outputs=[5 5]
  Display : Display
  Display1 : Display
  Display2 : Display
  Sonar trigger : Subsystem
  Subsystem : Subsystem
  Terminator : Terminator
  flag_sonar_func : MATLAB Function  TreatAsAtomicUnit=on
  Flag_sonar : Outport
  Rel_distance : Outport  Port=2
  Rel_angle : Outport  Port=3
  wires:
  Sonar trigger/1(Out2) -> Subsystem/Trigger
  Orientation/1 -> Subsystem/2(Orientation)
  Subsystem/1(Rel_distance) -> Rel_distance/1
  Subsystem/2(Rel_angle) -> Rel_angle/1
  Demux/1 -> Display2/1
  Demux/2 -> Display1/1
  flag_sonar_func/1(flag) -> Flag_sonar/1
  Sonar/1 -> Demux/1, Sonar trigger/1(In1), Demux1/1, Subsystem/1(Sonar)
  Demux1/1 -> Terminator/1
  Demux1/2 -> flag_sonar_func/1(flag_sonar)
  Subsystem/3(flag_sonar) -> Display/1

== system modello_completo_simulink2020/Navigation1/z_EKF ==
  meas_pos : Inport
  Depth_meas : Inport  Port=2
  ahrs_flag : Inport  Port=3
  orientation : Inport  Port=4
  dvl : Inport  Port=5
  Demux : Demux  Outputs=2
  Demux1 : Demux  Outputs=[2 1]
  Demux2 : Demux  Outputs=[2 1]
  Demux3 : Demux  Outputs=2
  EXTENDED KALMAN FILTER : Subsystem  TreatAsAtomicUnit=on
  Switch : Switch  Criteria=u2 ~= 0  RndMeth=Zero
  Terminator : Terminator
  Terminator1 : Terminator
  Trigger & Init : Subsystem
  Estimated position : Outport
  Estimation depth : Outport  Port=2
  flag_depth : Outport  Port=3
  wires:
  Trigger & Init/3(init) -> EXTENDED KALMAN FILTER/2(init)
  orientation/1 -> EXTENDED KALMAN FILTER/7(orientation)
  Demux2/2 -> EXTENDED KALMAN FILTER/5(GPS_flag)
  ahrs_flag/1 -> Demux1/1
  Trigger & Init/1(pulse) -> EXTENDED KALMAN FILTER/Trigger
  dvl/1 -> EXTENDED KALMAN FILTER/8(dvl)
  Trigger & Init/2(dT) -> EXTENDED KALMAN FILTER/1(dT)
  Trigger & Init/4(P0) -> EXTENDED KALMAN FILTER/3(P0)
  meas_pos/1 -> Demux2/1, Demux/1, Trigger & Init/2("meas_pos ")
  Demux1/1 -> Terminator/1
  Demux2/1 -> EXTENDED KALMAN FILTER/4(meas_pos)
  Demux1/2 -> EXTENDED KALMAN FILTER/9(ahrs_flag)
  Depth_meas/1 -> Trigger & Init/1(meas_depth), Demux3/1
  EXTENDED KALMAN FILTER/2(hat_depth) -> Estimation depth/1
  Demux/1 -> Switch/3
  EXTENDED KALMAN FILTER/1(hat_pos) -> Switch/1, Switch/2
  Switch/1 -> Estimated position/1
  Demux3/1 -> EXTENDED KALMAN FILTER/6(meas_depth)
  Demux3/2 -> flag_depth/1
  Demux/2 -> Terminator1/1

== system modello_completo_simulink2020/Vehicle Model/Manual (by dashboard sensors) ==
  Fx : Constant
  Fy : Constant  Value=0
  Fz : Constant  Value=0
  Mux2 : Mux  Inputs=6
  Pitch : Constant  Value=0
  Roll : Constant  Value=0
  Yaw : Constant  Value=0
  y : Outport
  wires:
  Fz/1 -> Mux2/3
  Fx/1 -> Mux2/1
  Yaw/1 -> Mux2/6
  Pitch/1 -> Mux2/5
  Fy/1 -> Mux2/2
  Roll/1 -> Mux2/4
  Mux2/1 -> y/1

== system modello_completo_simulink2020/Vehicle Model/Model Vehicle ==
  tau : Inport
  ni_current : Inport  Port=2
  Add : Sum  Inputs=+-+-
  Add1 : Sum  Inputs=|+-
  Add2 : Sum  Inputs=++|
  C : MATLAB Function  TreatAsAtomicUnit=on
  Constant1 : Constant  Value=rho
  Constant3 : Constant  Value=M
  Constant4 : Constant  Value=initial
  Constant5 : Constant  Value=pylonCenter
  D : MATLAB Function  TreatAsAtomicUnit=on
  Integrator : Integrator
  Integrator1 : Integrator
  Inversa di M : Constant  Value=M_inv
  Kinematic : Subsystem
      mask Display: image('$imagefile'); % Use "Edit Image" on toolstrip to change.
  MATLAB Function : MATLAB Function  TreatAsAtomicUnit=on
  Mux : Mux
  Product : Product  Multiplication=Matrix(*)
  grav : MATLAB Function  TreatAsAtomicUnit=on
  Out1 : Outport  VectorParamsAs1DForOutWhenUnconnected=off
  wires:
  tau/1 -> Add/1
  Product/1 -> Mux/4, Integrator/1  "ni_dot"
  Integrator/1 -> Kinematic/2(ni), Mux/3, Add1/1  "ni"
  ni_current/1 -> Add1/2
  Add1/1 -> D/1(ni_r), C/1(ni_r)  "ni_r"
  Mux/1 -> Out1/1
  C/1(F_c) -> Add/2  "F_c"
  grav/1(F_g) -> Add/4  "F_g"
  Kinematic/1(eta_dot) -> Mux/2, Integrator1/1  "eta_dot"
  Inversa di M/1 -> Product/1
  Add/1 -> Product/2  "M*ni_dot"
  Constant1/1 -> grav/1(rho), D/2(rho)
  Constant3/1 -> C/2(M)
  D/1(F_d) -> Add/3  "F_d"
  Add2/1 -> grav/2(eta), Kinematic/1(eta), MATLAB Function/2(eta)  "eta  3 - m 3 - rad"
  MATLAB Function/1(eta_ecef) -> Mux/1  "eta lat (deg) lon (deg) m 3 rad"
  Constant5/1 -> MATLAB Function/1(coord_pylon)
  Constant4/1 -> Add2/1
  Integrator1/1 -> Add2/2  "eta"

== system modello_completo_simulink2020/Vehicle Model/Thrusters ==
  des rot : Inport
  eta : Inport  Port=2
  ni : Inport  Port=3
  Product : Product  Multiplication=Matrix(*)
  T : Subsystem
      mask Display: image('$imagefile'); % Use "Edit Image" on toolstrip to change.
  TAM : Constant  Value=TAM
  saturation_tau : MATLAB Function  TreatAsAtomicUnit=on
  tau : Outport  VectorParamsAs1DForOutWhenUnconnected=off
  wires:
  Product/1 -> saturation_tau/1(tau)
  des rot/1 -> T/1(des rot)
  TAM/1 -> Product/1
  T/1(T) -> Product/2
  saturation_tau/1(tau_sat) -> tau/1
  ni/1 -> T/2(ni)
  eta/1 -> saturation_tau/2(eta)

== system modello_completo_simulink2020/Controller/AVVICINAMENTO/PID_HEAVE ==
  depth_err : Inport
  EN5 : Inport  Port=2
  Constant : Constant  Value=0
  Discrete-Time Integrator : DiscreteIntegrator  ExternalReset=falling  SampleTime=0.1  ICPrevOutput=DiscIntNeverNeededParam  ICPrevScaledInput=DiscIntNeverNeededParam
  Gain : Gain  Gain=Kp_depth2
  Gain2 : Gain  Gain=Ki_depth2
  Sum : Sum  Inputs=++|
  Switch : Switch  Criteria=u2 > Threshold  Threshold=0.5
  tau_depth : Outport
  wires:
  Gain/1 -> Sum/1
  Discrete-Time Integrator/1 -> Sum/2
  Constant/1 -> Switch/3
  Switch/1 -> Gain/1, Gain2/1
  depth_err/1 -> Switch/1
  Sum/1 -> tau_depth/1
  Gain2/1 -> Discrete-Time Integrator/1
  EN5/1 -> [EN5], Switch/2
  [EN5] -> Discrete-Time Integrator/2

== system modello_completo_simulink2020/Controller/AVVICINAMENTO/PID_PITCH ==
  pitch_err : Inport
  EN6 : Inport  Port=2
  Constant : Constant  Value=0
  Discrete-Time Integrator : DiscreteIntegrator  ExternalReset=falling  SampleTime=0.1  ICPrevOutput=DiscIntNeverNeededParam  ICPrevScaledInput=DiscIntNeverNeededParam
  Gain : Gain  Gain=Kp_P2
  Gain2 : Gain  Gain=Ki_P2
  Sum : Sum  Inputs=++|
  Switch : Switch  Criteria=u2 > Threshold  Threshold=0.5
  tau_pitch : Outport
  wires:
  [EN6] -> Discrete-Time Integrator/2
  Gain2/1 -> Discrete-Time Integrator/1
  Sum/1 -> tau_pitch/1
  Discrete-Time Integrator/1 -> Sum/2
  Gain/1 -> Sum/1
  pitch_err/1 -> Switch/1
  EN6/1 -> [EN6], Switch/2
  Constant/1 -> Switch/3
  Switch/1 -> Gain2/1, Gain/1

== system modello_completo_simulink2020/Controller/AVVICINAMENTO/PID_ROLL  ==
  roll_err : Inport
  EN6 : Inport  Port=2
  Constant : Constant  Value=0
  Discrete-Time Integrator : DiscreteIntegrator  ExternalReset=falling  SampleTime=0.1  ICPrevOutput=DiscIntNeverNeededParam  ICPrevScaledInput=DiscIntNeverNeededParam
  Gain : Gain  Gain=Kp_R2
  Gain2 : Gain  Gain=Ki_R2
  Sum : Sum  Inputs=++|
  Switch : Switch  Criteria=u2 > Threshold  Threshold=0.5
  tau_roll : Outport
  wires:
  Constant/1 -> Switch/3
  Discrete-Time Integrator/1 -> Sum/2
  Gain/1 -> Sum/1
  Gain2/1 -> Discrete-Time Integrator/1
  Sum/1 -> tau_roll/1
  roll_err/1 -> Switch/1
  EN6/1 -> [EN6], Switch/2
  Switch/1 -> Gain2/1, Gain/1
  [EN6] -> Discrete-Time Integrator/2

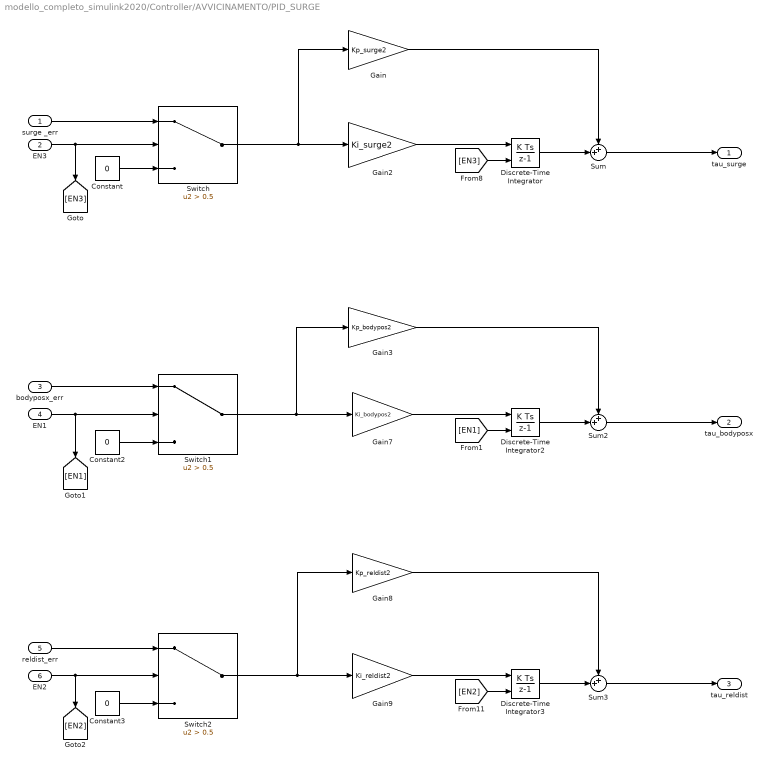
== system modello_completo_simulink2020/Controller/AVVICINAMENTO/PID_SURGE ==
  surge _err : Inport
  EN3 : Inport  Port=2
  bodyposx_err : Inport  Port=3
  EN1 : Inport  Port=4
  reldist_err : Inport  Port=5
  EN2 : Inport  Port=6
  Constant : Constant  Value=0
  Constant2 : Constant  Value=0
  Constant3 : Constant  Value=0
  Discrete-Time Integrator : DiscreteIntegrator  ExternalReset=falling  SampleTime=0.1  ICPrevOutput=DiscIntNeverNeededParam  ICPrevScaledInput=DiscIntNeverNeededParam
  Discrete-Time Integrator2 : DiscreteIntegrator  ExternalReset=falling  SampleTime=0.1  ICPrevOutput=DiscIntNeverNeededParam  ICPrevScaledInput=DiscIntNeverNeededParam
  Discrete-Time Integrator3 : DiscreteIntegrator  ExternalReset=falling  SampleTime=0.1  ICPrevOutput=DiscIntNeverNeededParam  ICPrevScaledInput=DiscIntNeverNeededParam
  Gain : Gain  Gain=Kp_surge2
  Gain2 : Gain  Gain=Ki_surge2
  Gain3 : Gain  Gain=Kp_bodypos2
  Gain7 : Gain  Gain=Ki_bodypos2
  Gain8 : Gain  Gain=Kp_reldist2
  Gain9 : Gain  Gain=Ki_reldist2
  Sum : Sum  Inputs=++|
  Sum2 : Sum  Inputs=++|
  Sum3 : Sum  Inputs=++|
  Switch : Switch  Criteria=u2 > Threshold  Threshold=0.5
  Switch1 : Switch  Criteria=u2 > Threshold  Threshold=0.5
  Switch2 : Switch  Criteria=u2 > Threshold  Threshold=0.5
  tau_surge : Outport
  tau_bodyposx : Outport  Port=2
  tau_reldist : Outport  Port=3
  wires:
  Gain/1 -> Sum/1
  Constant/1 -> Switch/3
  [EN3] -> Discrete-Time Integrator/2
  Discrete-Time Integrator/1 -> Sum/2
  Gain2/1 -> Discrete-Time Integrator/1
  Sum/1 -> tau_surge/1
  surge _err/1 -> Switch/1
  EN3/1 -> [EN3], Switch/2
  Switch/1 -> Gain2/1, Gain/1
  Gain7/1 -> Discrete-Time Integrator2/1
  Discrete-Time Integrator2/1 -> Sum2/2
  Gain3/1 -> Sum2/1
  Constant2/1 -> Switch1/3
  bodyposx_err/1 -> Switch1/1
  EN1/1 -> Switch1/2, [EN1]
  Switch1/1 -> Gain7/1, Gain3/1
  [EN1] -> Discrete-Time Integrator2/2
  Constant3/1 -> Switch2/3
  Gain8/1 -> Sum3/1
  Sum3/1 -> tau_reldist/1
  Switch2/1 -> Gain8/1, Gain9/1
  Discrete-Time Integrator3/1 -> Sum3/2
  [EN2] -> Discrete-Time Integrator3/2
  reldist_err/1 -> Switch2/1
  EN2/1 -> Switch2/2, [EN2]
  Gain9/1 -> Discrete-Time Integrator3/1
  Sum2/1 -> tau_bodyposx/1

== system modello_completo_simulink2020/Controller/AVVICINAMENTO/PID_SWAY ==
  latvel_err : Inport
  EN4 : Inport  Port=2
  bodyposy_err : Inport  Port=3
  EN1 : Inport  Port=4
  Constant : Constant  Value=0
  Constant1 : Constant  Value=0
  Discrete-Time Integrator : DiscreteIntegrator  ExternalReset=falling  SampleTime=0.1  ICPrevOutput=DiscIntNeverNeededParam  ICPrevScaledInput=DiscIntNeverNeededParam
  Discrete-Time Integrator1 : DiscreteIntegrator  ExternalReset=falling  SampleTime=0.1  ICPrevOutput=DiscIntNeverNeededParam  ICPrevScaledInput=DiscIntNeverNeededParam
  Gain : Gain  Gain=Kp_latvel2
  Gain1 : Gain  Gain=Kp_bodypos2
  Gain2 : Gain  Gain=Ki_latvel2
  Gain4 : Gain  Gain=Ki_bodypos2
  Sum : Sum  Inputs=++|
  Sum1 : Sum  Inputs=++|
  Switch : Switch  Criteria=u2 > Threshold  Threshold=0.5
  Switch1 : Switch  Criteria=u2 > Threshold  Threshold=0.5
  tau_latvel : Outport
  tau_bodyposy : Outport  Port=2
  wires:
  Constant/1 -> Switch/3
  Sum/1 -> tau_latvel/1
  Gain/1 -> Sum/1
  Switch/1 -> Gain/1, Gain2/1
  Discrete-Time Integrator/1 -> Sum/2
  Gain2/1 -> Discrete-Time Integrator/1
  latvel_err/1 -> Switch/1
  [EN4] -> Discrete-Time Integrator/2
  EN4/1 -> [EN4], Switch/2
  Discrete-Time Integrator1/1 -> Sum1/2
  Gain1/1 -> Sum1/1
  Gain4/1 -> Discrete-Time Integrator1/1
  [EN1] -> Discrete-Time Integrator1/2
  EN1/1 -> Switch1/2, [EN1]
  Constant1/1 -> Switch1/3
  bodyposy_err/1 -> Switch1/1
  Switch1/1 -> Gain1/1, Gain4/1
  Sum1/1 -> tau_bodyposy/1

== system modello_completo_simulink2020/Controller/AVVICINAMENTO/PID_YAW ==
  yaw_err : Inport
  "EN8 " : Inport  Port=2
  rel_or_err : Inport  Port=3
  EN7 : Inport  Port=4
  Constant : Constant  Value=0
  Constant1 : Constant  Value=0
  Discrete-Time Integrator : DiscreteIntegrator  ExternalReset=falling  SampleTime=0.1  ICPrevOutput=DiscIntNeverNeededParam  ICPrevScaledInput=DiscIntNeverNeededParam
  Discrete-Time Integrator1 : DiscreteIntegrator  ExternalReset=falling  SampleTime=0.1  ICPrevOutput=DiscIntNeverNeededParam  ICPrevScaledInput=DiscIntNeverNeededParam
  Gain : Gain  Gain=Kp_yaw2
  Gain1 : Gain  Gain=Kp_rel_or2
  Gain2 : Gain  Gain=Ki_yaw2
  Gain3 : Gain  Gain=Ki_rel_or2
  Sum : Sum  Inputs=++|
  Sum1 : Sum  Inputs=++|
  Switch : Switch  Criteria=u2 > Threshold  Threshold=0.5
  Switch1 : Switch  Criteria=u2 > Threshold  Threshold=0.5
  tau_yaw : Outport
  tau_rel_or : Outport  Port=2
  wires:
  Sum/1 -> tau_yaw/1
  Discrete-Time Integrator/1 -> Sum/2
  Switch/1 -> Gain/1, Gain2/1
  yaw_err/1 -> Switch/1
  Gain/1 -> Sum/1
  "EN8 "/1 -> [EN8], Switch/2
  Constant/1 -> Switch/3
  Gain2/1 -> Discrete-Time Integrator/1
  [EN8] -> Discrete-Time Integrator/2
  Discrete-Time Integrator1/1 -> Sum1/2
  [EN7] -> Discrete-Time Integrator1/2
  rel_or_err/1 -> Switch1/1
  EN7/1 -> [EN7], Switch1/2
  Switch1/1 -> Gain1/1, Gain3/1
  Sum1/1 -> tau_rel_or/1
  Constant1/1 -> Switch1/3
  Gain3/1 -> Discrete-Time Integrator1/1
  Gain1/1 -> Sum1/1

== system modello_completo_simulink2020/Controller/GEODETIC2NED2/GEODETIC2NED1 ==
  In1 : Inport
  Demux : Demux  Outputs=2
  MATLAB Function : MATLAB Function  TreatAsAtomicUnit=on
  Out1 : Outport
  wires:
  MATLAB Function/1(pos_s_Ned) -> Out1/1
  In1/1 -> Demux/1
  Demux/1 -> MATLAB Function/1(lat)
  Demux/2 -> MATLAB Function/2(lon)

== system modello_completo_simulink2020/Controller/GEODETIC2NED3/GEODETIC2NED ==
  lat : Inport  Unit=deg  PortDimensions=1
  lon : Inport  Port=2  Unit=deg  PortDimensions=1
  MATLAB Function : MATLAB Function  TreatAsAtomicUnit=on
  Out1 : Outport  Unit=m  PortDimensions=3
  wires:
  lat/1 -> MATLAB Function/1(lat)
  lon/1 -> MATLAB Function/2(lon)
  MATLAB Function/1(pos_Ned) -> Out1/1

== system modello_completo_simulink2020/Controller/IMMERSIONE//RISALITA/PID_HEAVE ==
  depth_err : Inport
  EN5 : Inport  Port=2
  Constant : Constant  Value=0
  Discrete-Time Integrator : DiscreteIntegrator  ExternalReset=falling  SampleTime=0.1  ICPrevOutput=DiscIntNeverNeededParam  ICPrevScaledInput=DiscIntNeverNeededParam
  Gain : Gain  Gain=Kp_depth4
  Gain2 : Gain  Gain=Ki_depth4
  Sum : Sum  Inputs=++|
  Switch : Switch  Criteria=u2 > Threshold  Threshold=0.5
  tau_depth : Outport
  wires:
  Gain/1 -> Sum/1
  Discrete-Time Integrator/1 -> Sum/2
  Constant/1 -> Switch/3
  Switch/1 -> Gain/1, Gain2/1
  depth_err/1 -> Switch/1
  Sum/1 -> tau_depth/1
  Gain2/1 -> Discrete-Time Integrator/1
  EN5/1 -> [EN5], Switch/2
  [EN5] -> Discrete-Time Integrator/2

== system modello_completo_simulink2020/Controller/IMMERSIONE//RISALITA/PID_PITCH ==
  pitch_err : Inport
  EN6 : Inport  Port=2
  Constant : Constant  Value=0
  Discrete-Time Integrator : DiscreteIntegrator  ExternalReset=falling  SampleTime=0.1  ICPrevOutput=DiscIntNeverNeededParam  ICPrevScaledInput=DiscIntNeverNeededParam
  Gain : Gain  Gain=Kp_P4
  Gain2 : Gain  Gain=Ki_P4
  Sum : Sum  Inputs=++|
  Switch : Switch  Criteria=u2 > Threshold  Threshold=0.5
  tau_pitch : Outport
  wires:
  [EN6] -> Discrete-Time Integrator/2
  Gain2/1 -> Discrete-Time Integrator/1
  Sum/1 -> tau_pitch/1
  Discrete-Time Integrator/1 -> Sum/2
  Gain/1 -> Sum/1
  pitch_err/1 -> Switch/1
  EN6/1 -> [EN6], Switch/2
  Constant/1 -> Switch/3
  Switch/1 -> Gain2/1, Gain/1

== system modello_completo_simulink2020/Controller/IMMERSIONE//RISALITA/PID_ROLL  ==
  roll_err : Inport
  EN6 : Inport  Port=2
  Constant : Constant  Value=0
  Discrete-Time Integrator : DiscreteIntegrator  ExternalReset=falling  SampleTime=0.1  ICPrevOutput=DiscIntNeverNeededParam  ICPrevScaledInput=DiscIntNeverNeededParam
  Gain : Gain  Gain=Kp_R4
  Gain2 : Gain  Gain=Ki_R4
  Sum : Sum  Inputs=++|
  Switch : Switch  Criteria=u2 > Threshold  Threshold=0.5
  tau_roll : Outport
  wires:
  Constant/1 -> Switch/3
  Discrete-Time Integrator/1 -> Sum/2
  Gain/1 -> Sum/1
  Gain2/1 -> Discrete-Time Integrator/1
  Sum/1 -> tau_roll/1
  roll_err/1 -> Switch/1
  EN6/1 -> [EN6], Switch/2
  Switch/1 -> Gain2/1, Gain/1
  [EN6] -> Discrete-Time Integrator/2

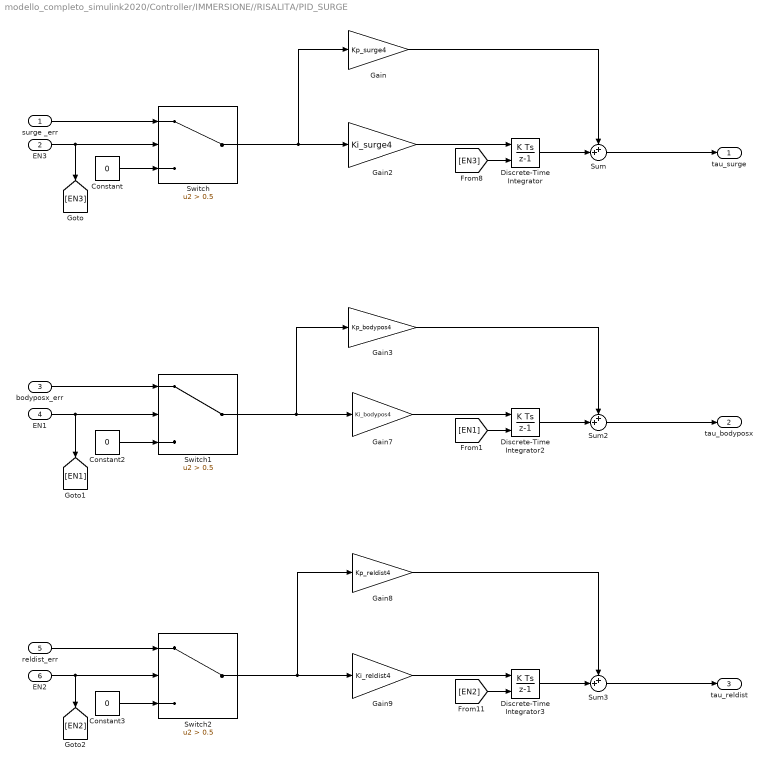
== system modello_completo_simulink2020/Controller/IMMERSIONE//RISALITA/PID_SURGE ==
  surge _err : Inport
  EN3 : Inport  Port=2
  bodyposx_err : Inport  Port=3
  EN1 : Inport  Port=4
  reldist_err : Inport  Port=5
  EN2 : Inport  Port=6
  Constant : Constant  Value=0
  Constant2 : Constant  Value=0
  Constant3 : Constant  Value=0
  Discrete-Time Integrator : DiscreteIntegrator  ExternalReset=falling  SampleTime=0.1  ICPrevOutput=DiscIntNeverNeededParam  ICPrevScaledInput=DiscIntNeverNeededParam
  Discrete-Time Integrator2 : DiscreteIntegrator  ExternalReset=falling  SampleTime=0.1  ICPrevOutput=DiscIntNeverNeededParam  ICPrevScaledInput=DiscIntNeverNeededParam
  Discrete-Time Integrator3 : DiscreteIntegrator  ExternalReset=falling  SampleTime=0.1  ICPrevOutput=DiscIntNeverNeededParam  ICPrevScaledInput=DiscIntNeverNeededParam
  Gain : Gain  Gain=Kp_surge4
  Gain2 : Gain  Gain=Ki_surge4
  Gain3 : Gain  Gain=Kp_bodypos4
  Gain7 : Gain  Gain=Ki_bodypos4
  Gain8 : Gain  Gain=Kp_reldist4
  Gain9 : Gain  Gain=Ki_reldist4
  Sum : Sum  Inputs=++|
  Sum2 : Sum  Inputs=++|
  Sum3 : Sum  Inputs=++|
  Switch : Switch  Criteria=u2 > Threshold  Threshold=0.5
  Switch1 : Switch  Criteria=u2 > Threshold  Threshold=0.5
  Switch2 : Switch  Criteria=u2 > Threshold  Threshold=0.5
  tau_surge : Outport
  tau_bodyposx : Outport  Port=2
  tau_reldist : Outport  Port=3
  wires:
  Gain/1 -> Sum/1
  Constant/1 -> Switch/3
  [EN3] -> Discrete-Time Integrator/2
  Discrete-Time Integrator/1 -> Sum/2
  Gain2/1 -> Discrete-Time Integrator/1
  Sum/1 -> tau_surge/1
  surge _err/1 -> Switch/1
  EN3/1 -> [EN3], Switch/2
  Switch/1 -> Gain2/1, Gain/1
  Gain7/1 -> Discrete-Time Integrator2/1
  Discrete-Time Integrator2/1 -> Sum2/2
  Gain3/1 -> Sum2/1
  Constant2/1 -> Switch1/3
  bodyposx_err/1 -> Switch1/1
  EN1/1 -> Switch1/2, [EN1]
  Switch1/1 -> Gain7/1, Gain3/1
  [EN1] -> Discrete-Time Integrator2/2
  Constant3/1 -> Switch2/3
  Gain8/1 -> Sum3/1
  Sum3/1 -> tau_reldist/1
  Switch2/1 -> Gain8/1, Gain9/1
  Discrete-Time Integrator3/1 -> Sum3/2
  [EN2] -> Discrete-Time Integrator3/2
  reldist_err/1 -> Switch2/1
  EN2/1 -> Switch2/2, [EN2]
  Gain9/1 -> Discrete-Time Integrator3/1
  Sum2/1 -> tau_bodyposx/1
